simulink model "sampleModel7"  (R2021a)
settings: Solver=VariableStepAuto  StartTime=0.0  StopTime=10.0  RelTol=1e-3
undefined symbols (not defined in the file): DiscIntNeverNeededParam, magnitude, Newton, Raphson
libraries: simulink x210, pid_lib x47, simulink_need_slupdate x2
(part 1 of 8)
settings Model: Creator=user  LastModifiedBy=user

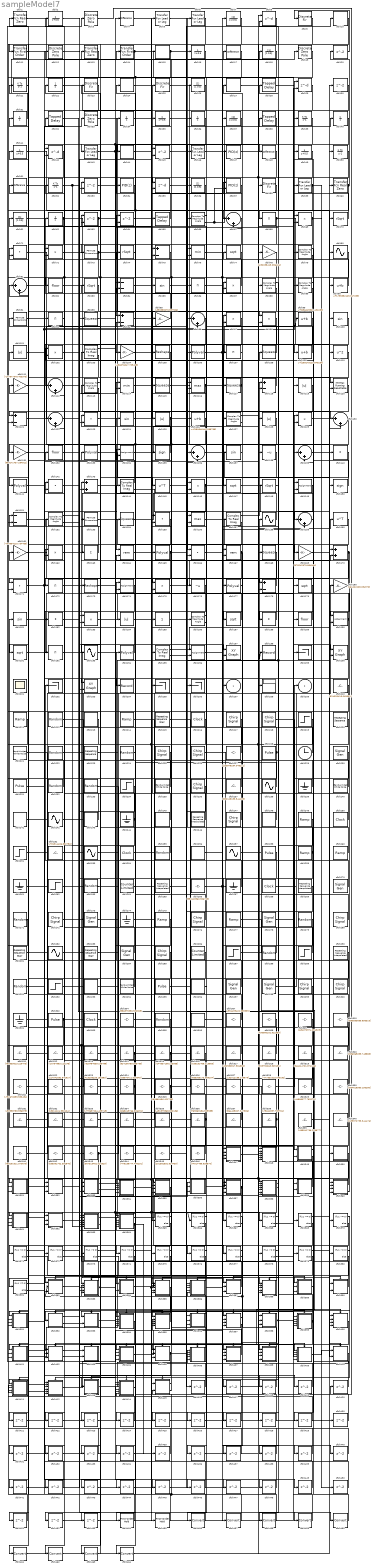
== system sampleModel7 ==
  cfblk1 : simulink/Discrete/Transfer Fcn Real Zero  ZeroZ=0.75  ICPrevInput=0.0  DoSatur=off
      settings: SourceProductBaseCode=SL
  cfblk{10,15,24,27,44} (5 alike) : DiscreteStateSpace
  cfblk{85,100,124,137,181} (5 alike) : Trigonometry
  cfblk{101,119,125,128,184} (5 alike) : Abs
  cfblk{69,98,102,162,175} (5 alike) : Product  Inputs=**
  cfblk{103,144,157,195} (4 alike) : ComplexToRealImag
  cfblk104 : Gain  Gain=[-436076047.709408]
  cfblk105 : Reshape
  cfblk{106,133,141,165,177,194} (6 alike) : Polyval  Coefs=[ +2.081618890e-019, -1.441693666e-014, +4.719686976e-010, -8.536869453e-006, +1.621573104e-001, -8.087801117e+001 ]
  cfblk{68,86,92,107,172,192} (6 alike) : Product  Inputs=*
  cfblk{93,108,115,117,154,168} (6 alike) : Squeeze
  cfblk109 : Bias  Bias=[299279220.840250]
  cfblk11 : simulink/Discrete/Transfer Fcn First Order  PoleZ=0.95  ICPrevOutput=0.0  DoSatur=off
  cfblk110 : Math  Operator=square  SaturateOnIntegerOverflow=on
  cfblk111 : Gain  Gain=[-177877978.403373]
  cfblk{67,81,96,112,122,130,136,139,159} (9 alike) : Sum  Inputs=|++
  cfblk{66,79,88..89,113,127,152,186} (8 alike) : ComplexToMagnitudeAngle
  cfblk114 : MinMax  Inputs=2
  cfblk116 : MinMax  Function=max  Inputs=2
  cfblk{75,94,118,121,178} (5 alike) : Sum  Inputs=+-
  cfblk{3,12,19,33} (4 alike) : DiscreteZeroPole  Poles=[0 0.5]  Gain=1
  cfblk120 : simulink/Math Operations/MinMax Running Resettable  Function=min  vinit=0.0
  cfblk{71,123,142,155,166,171} (6 alike) : DotProduct  InputSameDT=on  OutDataTypeStr=Inherit: Inherit via internal rule
  cfblk126 : Bias  Bias=[180646440.098758]
  cfblk{72,87,97,129,146,183} (6 alike) : Product
  cfblk13 : simulink/Discrete/Transfer Fcn Real Zero  ZeroZ=0.75  ICPrevInput=0.0  DoSatur=off
      settings: SourceProductBaseCode=SL
  cfblk131 : Gain  Gain=[934271437.284511]
  cfblk132 : Rounding
  cfblk{134,149,174,190,196} (5 alike) : Assignment  DiagnosticForDimensions=Warning  IndexOptions=Index vector (dialog)  Indices=1  OutputSizes=1
  cfblk135 : Signum
  cfblk138 : UnaryMinus
  cfblk14 : simulink/Discrete/Transfer Fcn First Order  PoleZ=0.95  ICPrevOutput=0.0  DoSatur=off
  cfblk{140,163,182,188} (4 alike) : Sum  Inputs=+
  cfblk143 : Sum
  cfblk145 : Math  Operator=transpose  SaturateOnIntegerOverflow=on
  cfblk{77,147,179,187,191} (5 alike) : Sqrt  SaturateOnIntegerOverflow=on
  cfblk{70,74,83,148} (4 alike) : Sqrt  Operator=rSqrt  AlgorithmType=Newton-Raphson  SaturateOnIntegerOverflow=on
  cfblk150 : Signum
  cfblk151 : Sum  Inputs=--
  cfblk153 : PermuteDimensions
  cfblk156 : MinMax  Function=max  Inputs=2
  cfblk158 : Sin  TimeSource=Use external signal  SampleTime=0
  cfblk{2,16,35,41,49} (5 alike) : DiscreteTransferFcn  SampleTime=1
  cfblk160 : Math  Operator=transpose  SaturateOnIntegerOverflow=on
  cfblk161 : Gain  Gain=[-744994210.734469]
  cfblk164 : Math  Operator=rem  SaturateOnIntegerOverflow=on
  cfblk167 : Math  Operator=rem  SaturateOnIntegerOverflow=on
  cfblk169 : Gain  Gain=[578242979.864904]
  cfblk{4,17,48,51} (4 alike) : simulink/Discrete/Difference  ICPrevInput=0.0  OutMin=[]  OutMax=[]  OutDataTypeStr=Inherit: Inherit via back propagation  OutDataType=fixdt(1, 16)  OutScaling=2^-10  DoSatur=off
  cfblk170 : Sum
  cfblk173 : Reshape
  cfblk176 : UnaryMinus
  cfblk{7,18,26,37,56,61} (6 alike) : DiscreteFilter  SampleTime=1
  cfblk180 : Gain  Gain=[161222208.054570]
  cfblk185 : simulink/Math Operations/Slider Gain  gain=1  low=0  high=2
  cfblk189 : Rounding
  cfblk193 : Sin  TimeSource=Use external signal  SampleTime=0
  cfblk197 : simulink/Sinks/XY Graph  xmin=-1  xmax=1  ymin=-1  ymax=1  st=-1
  cfblk198 : Record  FileSettingsInternal="{\"entries\":[{\"content\":{\"excelSettings\":{\"content\":{},\"type\":\"Streamout.ExcelSettings\"}},\"type\":\"Streamout.FileSettingStorage\",\"uuid\":\"33b5f820-dc1f-4b1a-ab87-c804d69286ae\"}],\"packageUris\":[\"http://schema.mathworks.com/mf0/streamout_blocks/R2020a\"],\"version\":\"1.0\"}"  SignalsInternal="{\"entries\":[{\"content\":{\"signals\":[{\"content\":{\"blockPath\":[\"sampleModel7/cfblk198\"],\"channel\":[],\"dimensions\":[1],\"domain\":\"samplemodel7/cfblk198\",\"lineColor\":\"#d95319\",\"plots\":[1],\"port\":1,\"sid\":[\"\"],\"signalID\":21002,\"signalName\":\"cfblk359\"},\"type\":\"RecordBlkView.Signal\",\"uuid\":\"796a8886-daab-4861-8312-900b38053f92\"}]},\"type\":\"RecordBlkView.InputSignals\",\"uuid\":\"0fedc28f-d636-42e2-b910-8174ae87f250\"}],\"packageUris\":[\"http://schema.mathworks.com/mf0/streamout_blocks/R2020a\"],\"version\":\"1.0\"}"  VisualizationBindings="{\"sparklinesplugin\":{\"info\":[{\"bindingParametersList\":[],\"subplotID\":1}]}}"
  cfblk{199,202,205..206} (4 alike) : Terminator
  cfblk{20,30,416..453} (40 alike) : Delay  SampleTime=1
  cfblk200 : simulink/Sinks/XY Graph  xmin=-1  xmax=1  ymin=-1  ymax=1  st=-1
  cfblk201 : Scope
      settings: Floating=on
  cfblk203 : simulink/Sinks/XY Graph  xmin=-1  xmax=1  ymin=-1  ymax=1  st=-1
  cfblk204 : Record  FileSettingsInternal="{\"entries\":[{\"content\":{\"excelSettings\":{\"content\":{},\"type\":\"Streamout.ExcelSettings\"}},\"type\":\"Streamout.FileSettingStorage\",\"uuid\":\"e6acbbf8-4b6b-4568-91b6-bdc9c77e83f1\"}],\"packageUris\":[\"http://schema.mathworks.com/mf0/streamout_blocks/R2020a\"],\"version\":\"1.0\"}"  SignalsInternal="{\"entries\":[{\"content\":{\"signals\":[{\"content\":{\"blockPath\":[\"sampleModel7/cfblk204\"],\"channel\":[],\"dimensions\":[1],\"domain\":\"samplemodel7/cfblk204\",\"lineColor\":\"#b746ff\",\"plots\":[1],\"port\":1,\"sid\":[\"\"],\"signalID\":21034,\"signalName\":\"cfblk26\"},\"type\":\"RecordBlkView.Signal\",\"uuid\":\"01d88a41-b529-4621-a6f8-95e57fe73dd8\"}]},\"type\":\"RecordBlkView.InputSignals\",\"uuid\":\"3bb34bcb-c099-496e-b3bc-84ef0106e8cb\"}],\"packageUris\":[\"http://schema.mathworks.com/mf0/streamout_blocks/R2020a\"],\"version\":\"1.0\"}"  VisualizationBindings="{\"sparklinesplugin\":{\"info\":[{\"bindingParametersList\":[],\"subplotID\":1}]}}"
  cfblk208 : Display
  cfblk{21,39,50,52} (4 alike) : DiscreteIntegrator  ICPrevOutput=DiscIntNeverNeededParam  ICPrevScaledInput=DiscIntNeverNeededParam
  cfblk210 : Constant  Value=[524020415.049531]  SampleTime=1
  cfblk211 : simulink/Sources/Ramp  slope=[1030.137133]  start=[45.427189]  InitialOutput=[816826.631031]
  cfblk212 : RandomNumber  Mean=[-9496.065728]  Variance=[4869.477426]  Seed=[748697780.000000]  SampleTime=0.1
  cfblk213 : simulink/Sources/Counter Free-Running  NumBits=[31.000000]  tsamp=-1
  cfblk214 : simulink/Sources/Ramp  slope=[-5450.476118]  start=[40.178251]  InitialOutput=[-351942.154890]
  cfblk215 : simulink/Sources/Repeating Sequence Stair  OutValues=[620097113.195074, 996961577.990435]  tsamp=-1  OutMin=[]  OutMax=[]  OutDataTypeStr=double  OutputDataTypeScalingMode=double  OutDataType=fixdt(0,8)  ConRadixGroup=Best Precision: Vector-wise  OutScaling=2^-12
  cfblk{216,250,254,268,303} (5 alike) : DigitalClock
  cfblk217 : simulink/Sources/Chirp Signal  f1=[743545607.434369]  T=[-343285056.387415]  f2=[305927425.208356]
  cfblk218 : simulink/Sources/Chirp Signal  f1=[-493852260.472383]  T=[857891074.645518]  f2=[-120015420.297469]
  cfblk219 : Step  Time=[26.000000]  Before=[-790798293.471162]  After=[399582314.918579]  SampleTime=0
  cfblk{22,31,34,36,40,62} (6 alike) : UnitDelay  HasFrameUpgradeWarning=on
  cfblk220 : simulink/Sources/Repeating Sequence  rep_seq_t=[0 2]  rep_seq_y=[213258458.389968, 48619559.079898]
  cfblk221 : simulink/Sources/Band-Limited White Noise  Cov=[6528417402.634652]  Ts=0.1  seed=[9893385339.000000]
  cfblk222 : RandomNumber  Mean=[59096.277871]  Variance=[64433.860844]  Seed=[883947103.000000]  SampleTime=0.1
  cfblk223 : simulink/Sources/Repeating Sequence  rep_seq_t=[0 2]  rep_seq_y=[-569792071.335092, -150840341.118165]
  cfblk224 : RandomNumber  Mean=[93987.666809]  Variance=[65814.423769]  Seed=[597783153.000000]  SampleTime=0.1
  cfblk225 : simulink/Sources/Chirp Signal  f1=[-378273320.468828]  T=[-983632335.403246]  f2=[969737135.267250]
  cfblk226 : simulink/Sources/Chirp Signal  f1=[-563170031.250757]  T=[464970760.325772]  f2=[602740179.436445]
  cfblk227 : Constant  Value=[200978294.048211]  SampleTime=1
  cfblk228 : DiscretePulseGenerator  PulseType=Time based  Amplitude=[-669665441.401893]  Period=[35025367.756640]  PulseWidth=5  PhaseDelay=[7.000000]
  cfblk229 : Clock
  cfblk{9,23,25,58} (4 alike) : DiscreteFir  SampleTime=1
  cfblk230 : SignalGenerator  Amplitude=[-992086751.304337]
  cfblk231 : DiscretePulseGenerator  PulseType=Time based  Amplitude=[984993340.582845]  Period=[36116761.892017]  PulseWidth=5  PhaseDelay=[3.000000]
  cfblk232 : UniformRandomNumber  Minimum=[-3818046436.640810]  Maximum=[5090086403.133304]  Seed=[56812594.000000]  SampleTime=0.1
  cfblk233 : UniformRandomNumber  Minimum=[-932888726.507126]  Maximum=[6609210111.863044]  Seed=[78621193.000000]  SampleTime=0.1
  cfblk234 : Step  Time=[14.000000]  Before=[-635477653.074702]  After=[674226947.834275]  SampleTime=0
  cfblk235 : simulink/Sources/Band-Limited White Noise  Cov=[491962027.885377]  Ts=0.1  seed=[1309214404.000000]
  cfblk236 : simulink/Sources/Chirp Signal  f1=[-403885962.803883]  T=[132909770.054147]  f2=[-111427795.279473]
  cfblk237 : Constant  Value=[852128153.544189]  SampleTime=1
  cfblk238 : Sin  Amplitude=[202876391.396995]  Bias=[622083626.491215]  SampleTime=0
  cfblk{239,244,261,267,274,301} (6 alike) : Ground
  cfblk240 : simulink/Sources/Band-Limited White Noise  Cov=[8151406213.355165]  Ts=0.1  seed=[616741273.000000]
  cfblk241 : simulink/Sources/Counter Free-Running  NumBits=[13.000000]  tsamp=-1
  cfblk242 : Sin  Amplitude=[-301429893.411587]  Bias=[-578206961.244922]  SampleTime=0
  cfblk243 : simulink/Sources/Counter Free-Running  NumBits=[13.000000]  tsamp=-1
  cfblk245 : simulink/Sources/Counter Free-Running  NumBits=[20.000000]  tsamp=-1
  cfblk246 : simulink/Sources/Repeating Sequence Interpolated  OutValues=[-450645048.681899, 465095687.906340, 414797516.535470, -426302903.466728, -987112265.543416]  TimeValues=[0 0.1 0.5 0.6 1].'  LookUpMeth=Use Input Nearest  tsamp=0.01  OutMin=[]  OutMax=[]  OutDataTypeStr=double  OutputDataTypeScalingMode=double  OutDataType=fixdt(0,8)  OutScaling=2^-10
  cfblk247 : simulink/Sources/Chirp Signal  f1=[-319865348.200507]  T=[-112136263.341765]  f2=[-601953811.778989]
  cfblk248 : simulink/Sources/Counter Free-Running  NumBits=[22.000000]  tsamp=-1
  cfblk249 : simulink/Sources/Ramp  slope=[4946.348764]  start=[16.631799]  InitialOutput=[956548.997204]
  cfblk251 : Step  Time=[48.000000]  Before=[695171433.417736]  After=[177666728.297122]  SampleTime=0
  cfblk252 : Constant  Value=[-781314406.882750]  SampleTime=1
  cfblk253 : Sin  Amplitude=[-11513605.676250]  Bias=[-821857418.853351]  SampleTime=0
  cfblk255 : UniformRandomNumber  Minimum=[-701801758.865852]  Maximum=[8678339802.126019]  Seed=[68934056.000000]  SampleTime=0.1
  cfblk256 : simulink/Sources/Counter Free-Running  NumBits=[19.000000]  tsamp=-1
  cfblk257 : Sin  Amplitude=[-411844016.363689]  Bias=[201928634.661419]  SampleTime=0
  cfblk258 : DiscretePulseGenerator  PulseType=Time based  Amplitude=[-474102356.549540]  Period=[30790102.267686]  PulseWidth=5  PhaseDelay=[3.000000]
  cfblk259 : simulink/Sources/Ramp  slope=[7960.944092]  start=[45.974135]  InitialOutput=[34137.177762]
  cfblk260 : simulink/Sources/Ramp  slope=[-104.563983]  start=[44.144888]  InitialOutput=[232608.767387]
  cfblk262 : Step  Time=[8.000000]  Before=[-777670275.272579]  After=[-705023258.616207]  SampleTime=0
  cfblk263 : RandomNumber  Mean=[92822.716429]  Variance=[49071.021235]  Seed=[630192977.000000]  SampleTime=0.1
  cfblk264 : simulink/Sources/Counter Limited  uplimit=[395.000000]  tsamp=-1
  cfblk265 : simulink/Sources/Repeating Sequence Interpolated  OutValues=[582550086.818798, 378877582.389652, 420436919.398782, -767860329.071510, 871635005.758899]  TimeValues=[0 0.1 0.5 0.6 1].'  LookUpMeth=Use Input Nearest  tsamp=0.01  OutMin=[]  OutMax=[]  OutDataTypeStr=double  OutputDataTypeScalingMode=double  OutDataType=fixdt(0,8)  OutScaling=2^-10
  cfblk266 : Constant  Value=[953418960.906703]  SampleTime=1
  cfblk269 : simulink/Sources/Repeating Sequence Interpolated  OutValues=[24439926.283149, -764111606.177588, 284652558.125769, -333748133.871525, 968266300.835480]  TimeValues=[0 0.1 0.5 0.6 1].'  LookUpMeth=Use Input Above  tsamp=0.01  OutMin=[]  OutMax=[]  OutDataTypeStr=double  OutputDataTypeScalingMode=double  OutDataType=fixdt(0,8)  OutScaling=2^-10
  cfblk270 : SignalGenerator  Amplitude=[894529370.076149]  Units=rad/sec
  cfblk271 : RandomNumber  Mean=[-87458.014011]  Variance=[15420.417994]  Seed=[930721984.000000]  SampleTime=0.1
  cfblk272 : simulink/Sources/Chirp Signal  f1=[-329172158.501780]  T=[-335641080.512788]  f2=[-39141377.640128]
  cfblk273 : SignalGenerator  WaveForm=square  Amplitude=[394650273.027109]  Units=rad/sec
  cfblk275 : simulink/Sources/Ramp  slope=[7083.231616]  start=[44.227960]  InitialOutput=[737333.840451]
  cfblk276 : simulink/Sources/Chirp Signal  f1=[-651584684.508423]  T=[-556322214.516704]  f2=[-126128626.986041]
  cfblk277 : simulink/Sources/Ramp  slope=[-9076.234007]  start=[31.699292]  InitialOutput=[-816121.492388]
  cfblk278 : SignalGenerator  WaveForm=square  Amplitude=[151893873.336181]
  cfblk279 : RandomNumber  Mean=[-86026.753652]  Variance=[87554.267207]  Seed=[329952460.000000]  SampleTime=0.1
  cfblk{28,32,38,65} (4 alike) : simulink/Discrete/Tapped Delay  vinit=0.0  samptime=-1  NumDelays=1  DelayOrder=Oldest  includeCurrent=off
  cfblk280 : simulink/Sources/Chirp Signal  f1=[903993729.853343]  T=[819500778.137060]  f2=[913581693.425247]
  cfblk281 : simulink/Sources/Repeating Sequence Stair  OutValues=[-518754567.655191, -580569798.246538]  tsamp=-1  OutMin=[]  OutMax=[]  OutDataTypeStr=double  OutputDataTypeScalingMode=double  OutDataType=fixdt(0,8)  ConRadixGroup=Best Precision: Vector-wise  OutScaling=2^-12
  cfblk282 : Sin  Amplitude=[5735855.369506]  Bias=[68993685.687378]  SampleTime=0
  cfblk283 : simulink/Sources/Repeating Sequence Stair  OutValues=[-908322828.357433, -917374741.295317]  tsamp=-1  OutMin=[]  OutMax=[]  OutDataTypeStr=double  OutputDataTypeScalingMode=double  OutDataType=fixdt(0,8)  ConRadixGroup=Best Precision: Vector-wise  OutScaling=2^-12
  cfblk284 : SignalGenerator  WaveForm=square  Amplitude=[526675952.966053]
  cfblk285 : simulink/Sources/Chirp Signal  f1=[193150470.797075]  T=[57635887.761176]  f2=[912894724.060447]
  cfblk286 : simulink/Sources/Counter Limited  uplimit=[404.000000]  tsamp=-1
  cfblk287 : Step  Time=[40.000000]  Before=[996055666.687662]  After=[251563225.588835]  SampleTime=0
  cfblk288 : UniformRandomNumber  Minimum=[-7496835967.641567]  Maximum=[8729181639.729187]  Seed=[5649486.000000]  SampleTime=0.1
  cfblk289 : Step  Time=[10.000000]  Before=[857137299.471670]  After=[-96536403.778174]  SampleTime=0
  cfblk{8,29,42,55} (4 alike) : Delay  DelayLengthSource=Input port  SampleTime=1
      settings: InputPortMap=u0,p1
  cfblk290 : simulink/Sources/Repeating Sequence Interpolated  OutValues=[565215223.963382, -475259355.929744, 977523137.003072, 200937123.605233, -160039889.164123]  TimeValues=[0 0.1 0.5 0.6 1].'  LookUpMeth=Use Input Above  tsamp=0.01  OutMin=[]  OutMax=[]  OutDataTypeStr=double  OutputDataTypeScalingMode=double  OutDataType=fixdt(0,8)  OutScaling=2^-10
  cfblk291 : RandomNumber  Mean=[-26763.666049]  Variance=[58579.543437]  Seed=[178776162.000000]  SampleTime=0.1
  cfblk292 : Step  Time=[30.000000]  Before=[116319489.559848]  After=[164052589.890091]  SampleTime=0
  cfblk293 : simulink/Sources/Counter Free-Running  NumBits=[21.000000]  tsamp=-1
  cfblk294 : simulink/Sources/Band-Limited White Noise  Cov=[1934120681.365680]  Ts=0.1  seed=[5475971794.000000]
  cfblk295 : DiscretePulseGenerator  PulseType=Time based  Amplitude=[596723854.655416]  Period=[36879074.032624]  PulseWidth=5  PhaseDelay=[5.000000]
  cfblk296 : simulink/Sources/Counter Free-Running  NumBits=[53.000000]  tsamp=-1
  cfblk297 : SignalGenerator  WaveForm=sawtooth  Amplitude=[656379074.653439]
  cfblk298 : SignalGenerator  Amplitude=[-439043768.529233]  Units=rad/sec
  cfblk299 : simulink/Sources/Chirp Signal  f1=[-753347408.556282]  T=[379872310.866754]  f2=[-968584085.001590]
  cfblk300 : simulink/Sources/Chirp Signal  f1=[604165645.787270]  T=[-503021265.049175]  f2=[819974698.514872]
  cfblk302 : DiscretePulseGenerator  PulseType=Time based  Amplitude=[-464926827.343680]  Period=[95246281.630336]  PulseWidth=5  PhaseDelay=[4.000000]
  cfblk304 : Constant  Value=[586575390.552825]  SampleTime=1
  cfblk305 : RandomNumber  Mean=[33528.370879]  Variance=[26957.875777]  Seed=[805936811.000000]  SampleTime=0.1
  cfblk306 : simulink/Sources/Counter Free-Running  NumBits=[53.000000]  tsamp=-1
  cfblk307 : Constant  Value=[-954439422.989939]  SampleTime=1
  cfblk308 : Constant  Value=[436080102.912559]  SampleTime=1
  cfblk309 : Constant  Value=[-634072574.054325]  SampleTime=1
  cfblk310 : Constant  Value=[-680553689.856316]  SampleTime=1
  cfblk311 : Constant  Value=[760535013.226473]  SampleTime=1
  cfblk312 : Constant  Value=[-16794983.122245]  SampleTime=1
  cfblk313 : Constant  Value=[-318484039.166498]  SampleTime=1
  cfblk314 : Constant  Value=[824106789.505750]  SampleTime=1
  cfblk315 : Constant  Value=[-244337108.123065]  SampleTime=1
  cfblk316 : Constant  Value=[-109231408.213983]  SampleTime=1
  cfblk317 : Constant  Value=[492980817.584880]  SampleTime=1
  cfblk318 : Constant  Value=[333792263.325191]  SampleTime=1
  cfblk319 : Constant  Value=[346214701.871126]  SampleTime=1
  cfblk320 : Constant  Value=[-956365099.748888]  SampleTime=1
  cfblk321 : Constant  Value=[-752670059.933454]  SampleTime=1
  cfblk322 : Constant  Value=[227041692.841627]  SampleTime=1
  cfblk323 : Constant  Value=[423295235.193383]  SampleTime=1
  cfblk324 : Constant  Value=[-35970711.013645]  SampleTime=1
  cfblk325 : Constant  Value=[-60860456.421755]  SampleTime=1
  cfblk326 : Constant  Value=[-665306173.089104]  SampleTime=1
  cfblk327 : Constant  Value=[132012188.179679]  SampleTime=1
  cfblk328 : Constant  Value=[-777531019.049252]  SampleTime=1
  cfblk329 : Constant  Value=[-44886077.763270]  SampleTime=1
  cfblk330 : Constant  Value=[-564618580.156280]  SampleTime=1
  cfblk331 : Constant  Value=[-58998783.596879]  SampleTime=1
  cfblk332 : Constant  Value=[15011124.930104]  SampleTime=1
  cfblk333 : Constant  Value=[-775637204.439745]  SampleTime=1
  cfblk334 : Constant  Value=[-868249766.306151]  SampleTime=1
  cfblk335 : Constant  Value=[-491979568.832186]  SampleTime=1
  cfblk336 : Constant  Value=[769063186.505985]  SampleTime=1
  cfblk337 : Constant  Value=[864425027.347386]  SampleTime=1
  cfblk338 : Constant  Value=[-75611897.789784]  SampleTime=1
  cfblk339 : Constant  Value=[-495541796.229877]  SampleTime=1
  cfblk340 : Constant  Value=[-159372753.344476]  SampleTime=1
  cfblk341 : Constant  Value=[765291611.070670]  SampleTime=1
  cfblk342 : Constant  Value=[635591702.392840]  SampleTime=1
  cfblk343 : Constant  Value=[367315462.010529]  SampleTime=1
  cfblk344 : Constant  Value=[-476238774.440251]  SampleTime=1
  cfblk345 : Constant  Value=[201382552.814439]  SampleTime=1
  cfblk346 : Constant  Value=[74017486.635570]  SampleTime=1
  cfblk347 : Subsystem
  cfblk348 : Subsystem
  cfblk349 : Subsystem
  cfblk350 : Subsystem
  cfblk351 : Subsystem
  cfblk352 : Subsystem
  cfblk353 : Subsystem
  cfblk354 : Subsystem
  cfblk355 : Subsystem
  cfblk356 : Subsystem
  cfblk357 : Subsystem
  cfblk358 : Subsystem
  cfblk359 : Subsystem
  cfblk360 : Subsystem
  cfblk361 : Subsystem
  cfblk362 : Subsystem
  cfblk363 : Subsystem
  cfblk364 : Subsystem
  cfblk{365..381} (17 alike) : If  IfExpression=u1 >= 0  SampleTime=1
  cfblk382 : Subsystem  TreatAsAtomicUnit=on
  cfblk383 : Subsystem  TreatAsAtomicUnit=on
  cfblk384 : Subsystem  TreatAsAtomicUnit=on
  cfblk385 : Subsystem  TreatAsAtomicUnit=on
  cfblk386 : Subsystem  TreatAsAtomicUnit=on
  cfblk387 : Subsystem  TreatAsAtomicUnit=on
  cfblk388 : Subsystem  TreatAsAtomicUnit=on
  cfblk389 : Subsystem  TreatAsAtomicUnit=on
  cfblk390 : Subsystem  TreatAsAtomicUnit=on
  cfblk391 : Subsystem  TreatAsAtomicUnit=on
  cfblk392 : Subsystem  TreatAsAtomicUnit=on
  cfblk393 : Subsystem  TreatAsAtomicUnit=on
  cfblk394 : Subsystem  TreatAsAtomicUnit=on
  cfblk395 : Subsystem  TreatAsAtomicUnit=on
  cfblk396 : Subsystem  TreatAsAtomicUnit=on
  cfblk397 : Subsystem  TreatAsAtomicUnit=on
  cfblk398 : Subsystem  TreatAsAtomicUnit=on
  cfblk399 : Subsystem  TreatAsAtomicUnit=on
  cfblk400 : Subsystem  TreatAsAtomicUnit=on
  cfblk401 : Subsystem  TreatAsAtomicUnit=on
  cfblk402 : Subsystem  TreatAsAtomicUnit=on
  cfblk403 : Subsystem  TreatAsAtomicUnit=on
  cfblk404 : Subsystem  TreatAsAtomicUnit=on
  cfblk405 : Subsystem  TreatAsAtomicUnit=on
  cfblk406 : Subsystem  TreatAsAtomicUnit=on
  cfblk407 : Subsystem  TreatAsAtomicUnit=on
  cfblk408 : Subsystem  TreatAsAtomicUnit=on
  cfblk409 : Subsystem  TreatAsAtomicUnit=on
  cfblk410 : Subsystem  TreatAsAtomicUnit=on
  cfblk411 : Subsystem  TreatAsAtomicUnit=on
  cfblk412 : Subsystem  TreatAsAtomicUnit=on
  cfblk413 : Subsystem  TreatAsAtomicUnit=on
  cfblk414 : Subsystem  TreatAsAtomicUnit=on
  cfblk415 : Subsystem  TreatAsAtomicUnit=on
  cfblk{5..6,43,46,59} (5 alike) : simulink/Discrete/Transfer Fcn Lead or Lag  PoleZ=0.95  ZeroZ=0.75  ICPrevOutput=0.0  ICPrevInput=0.0  DoSatur=off
      settings: SourceProductBaseCode=SL
  cfblk{45,53,63..64} (4 alike) : Delay  ShowEnablePort=on  SampleTime=1
      settings: InputPortMap=u0,e6
  cfblk454 : simulink_need_slupdate/First-Order Hold  DisableCoverage=on  Ts=1
      settings: SourceProductBaseCode=SL
  cfblk455 : simulink_need_slupdate/First-Order Hold  DisableCoverage=on  Ts=1
      settings: SourceProductBaseCode=SL
  cfblk{456..464} (9 alike) : DataTypeConversion
  cfblk47 : pid_lib/PID Controller  Controller=PID  Form=Parallel  TimeDomain=Discrete-time  UseExternalTs=off  SampleTime=1  IntegratorMethod=Forward Euler  FilterMethod=Forward Euler  ControllerParametersSource=internal  P=1  I=1  D=0  UseFilter=on  N=100  TunerSelectOption=Transfer Function Based (PID Tuner App)  InitialConditionSource=internal  InitialConditionForIntegrator=0  InitialConditionForFilter=0  DifferentiatorICPrevScaledInput=0  ExternalReset=none  TrackingMode=off  Kt=1  LimitOutput=off  SatLimitsSource=internal  UpperSaturationLimit=inf  LowerSaturationLimit=-inf  LinearizeAsGain=off  AntiWindupMode=none  Kb=1  POutMin=[]  POutMax=[]  IOutMin=[]  IOutMax=[]  DOutMin=[]  DOutMax=[]  NOutMin=[]  NOutMax=[]  SumOutMin=[]  SumOutMax=[]  SaturationOutMin=[]  SaturationOutMax=[]  PParamMin=[]  PParamMax=[]  IParamMin=[]  IParamMax=[]  DParamMin=[]  DParamMax=[]  NParamMin=[]  NParamMax=[]  KbParamMin=[]  KbParamMax=[]  KtParamMin=[]  KtParamMax=[]  KbOutMin=[]  KbOutMax=[]  KtOutMin=[]  KtOutMax=[]  IntegratorOutMin=[]  IntegratorOutMax=[]  FilterOutMin=[]  FilterOutMax=[]  SumI1OutMin=[]  SumI1OutMax=[]  SumI2OutMin=[]  SumI2OutMax=[]  SumI3OutMin=[]  SumI3OutMax=[]  SumI4OutMin=[]  SumI4OutMax=[]  SumDOutMin=[]  SumDOutMax=[]  DifferentiatorOutMin=[]  DifferentiatorOutMax=[]  FilterDiffOutCoefMin=[]  FilterDiffOutCoefMax=[]  ReciprocalOutMin=[]  ReciprocalOutMax=[]  SumDenOutMin=[]  SumDenOutMax=[]  SumNumOutMin=[]  SumNumOutMax=[]  DivideOutMin=[]  DivideOutMax=[]  UdiffTsProdOutMin=[]  UdiffTsProdOutMax=[]  NTsProdOutMin=[]  NTsProdOutMax=[]  UintegralTsProdOutMin=[]  UintegralTsProdOutMax=[]  UngainTsProdOutMin=[]  UngainTsProdOutMax=[]  IntegratorContinuousStateAttributes=''  IntegratorStateMustResolveToSignalObject=off  IntegratorRTWStateStorageClass=Auto  FilterContinuousStateAttributes=''  FilterStateMustResolveToSignalObject=off  FilterRTWStateStorageClass=Auto  ParallelPVariant=InternalParameters  IdealPVariant=Disabled  IVariant=InternalParameters  DVariant=InternalParameters  IntegratorVariant=Discrete  SatVariant=Disabled  AWVariant=Passthrough  PCopyVariant=Disabled  TRVariant=Disabled  FdbkBlocksVariant=Forward  IdealPFdbkVariant=Disabled  SatFdbkVariant=Disabled  DerivativeFilterVariant=ForwardEulerFilter  NVariant=InternalParameters  NCopyVariant=Disabled  FilterICVariant=InternalICsFilter  IntegratorICVariant=InternalICs  ExternalResetVariant=Disabled  TRSumVariant=Passthrough  SumFdbkVariant=Disabled  SumVariant=Sum_PID  TsampFilterVariant=InternalTs  TsampNgainVariant=Passthrough  TsampIntegralVariant=Passthrough  ExternalSaturationOutDataTypeStr=Inherit: Same as second input
  cfblk54 : pid_lib/PID Controller  Controller=PID  Form=Parallel  TimeDomain=Discrete-time  UseExternalTs=off  SampleTime=1  IntegratorMethod=Forward Euler  FilterMethod=Forward Euler  ControllerParametersSource=internal  P=1  I=1  D=0  UseFilter=on  N=100  TunerSelectOption=Transfer Function Based (PID Tuner App)  InitialConditionSource=internal  InitialConditionForIntegrator=0  InitialConditionForFilter=0  DifferentiatorICPrevScaledInput=0  ExternalReset=none  TrackingMode=off  Kt=1  LimitOutput=off  SatLimitsSource=internal  UpperSaturationLimit=inf  LowerSaturationLimit=-inf  LinearizeAsGain=off  AntiWindupMode=none  Kb=1  POutMin=[]  POutMax=[]  IOutMin=[]  IOutMax=[]  DOutMin=[]  DOutMax=[]  NOutMin=[]  NOutMax=[]  SumOutMin=[]  SumOutMax=[]  SaturationOutMin=[]  SaturationOutMax=[]  PParamMin=[]  PParamMax=[]  IParamMin=[]  IParamMax=[]  DParamMin=[]  DParamMax=[]  NParamMin=[]  NParamMax=[]  KbParamMin=[]  KbParamMax=[]  KtParamMin=[]  KtParamMax=[]  KbOutMin=[]  KbOutMax=[]  KtOutMin=[]  KtOutMax=[]  IntegratorOutMin=[]  IntegratorOutMax=[]  FilterOutMin=[]  FilterOutMax=[]  SumI1OutMin=[]  SumI1OutMax=[]  SumI2OutMin=[]  SumI2OutMax=[]  SumI3OutMin=[]  SumI3OutMax=[]  SumI4OutMin=[]  SumI4OutMax=[]  SumDOutMin=[]  SumDOutMax=[]  DifferentiatorOutMin=[]  DifferentiatorOutMax=[]  FilterDiffOutCoefMin=[]  FilterDiffOutCoefMax=[]  ReciprocalOutMin=[]  ReciprocalOutMax=[]  SumDenOutMin=[]  SumDenOutMax=[]  SumNumOutMin=[]  SumNumOutMax=[]  DivideOutMin=[]  DivideOutMax=[]  UdiffTsProdOutMin=[]  UdiffTsProdOutMax=[]  NTsProdOutMin=[]  NTsProdOutMax=[]  UintegralTsProdOutMin=[]  UintegralTsProdOutMax=[]  UngainTsProdOutMin=[]  UngainTsProdOutMax=[]  IntegratorContinuousStateAttributes=''  IntegratorStateMustResolveToSignalObject=off  IntegratorRTWStateStorageClass=Auto  FilterContinuousStateAttributes=''  FilterStateMustResolveToSignalObject=off  FilterRTWStateStorageClass=Auto  ParallelPVariant=InternalParameters  IdealPVariant=Disabled  IVariant=InternalParameters  DVariant=InternalParameters  IntegratorVariant=Discrete  SatVariant=Disabled  AWVariant=Passthrough  PCopyVariant=Disabled  TRVariant=Disabled  FdbkBlocksVariant=Forward  IdealPFdbkVariant=Disabled  SatFdbkVariant=Disabled  DerivativeFilterVariant=ForwardEulerFilter  NVariant=InternalParameters  NCopyVariant=Disabled  FilterICVariant=InternalICsFilter  IntegratorICVariant=InternalICs  ExternalResetVariant=Disabled  TRSumVariant=Passthrough  SumFdbkVariant=Disabled  SumVariant=Sum_PID  TsampFilterVariant=InternalTs  TsampNgainVariant=Passthrough  TsampIntegralVariant=Passthrough  ExternalSaturationOutDataTypeStr=Inherit: Same as second input
  cfblk57 : pid_lib/PID Controller (2DOF)  Controller=PID  Form=Parallel  TimeDomain=Discrete-time  UseExternalTs=off  SampleTime=1  IntegratorMethod=Forward Euler  FilterMethod=Forward Euler  ControllerParametersSource=internal  P=1  I=1  D=0  UseFilter=on  N=100  b=1  c=1  TunerSelectOption=Transfer Function Based (PID Tuner App)  InitialConditionSource=internal  InitialConditionForIntegrator=0  InitialConditionForFilter=0  DifferentiatorICPrevScaledInput=0  ExternalReset=none  TrackingMode=off  Kt=1  LimitOutput=off  SatLimitsSource=internal  UpperSaturationLimit=inf  LowerSaturationLimit=-inf  LinearizeAsGain=off  AntiWindupMode=none  Kb=1  POutMin=[]  POutMax=[]  IOutMin=[]  IOutMax=[]  DOutMin=[]  DOutMax=[]  NOutMin=[]  NOutMax=[]  bOutMin=[]  bOutMax=[]  cOutMin=[]  cOutMax=[]  SumOutMin=[]  SumOutMax=[]  SaturationOutMin=[]  SaturationOutMax=[]  PParamMin=[]  PParamMax=[]  IParamMin=[]  IParamMax=[]  DParamMin=[]  DParamMax=[]  NParamMin=[]  NParamMax=[]  bParamMin=[]  bParamMax=[]  cParamMin=[]  cParamMax=[]  KbParamMin=[]  KbParamMax=[]  KtParamMin=[]  KtParamMax=[]  KbOutMin=[]  KbOutMax=[]  KtOutMin=[]  KtOutMax=[]  IntegratorOutMin=[]  IntegratorOutMax=[]  FilterOutMin=[]  FilterOutMax=[]  SumI1OutMin=[]  SumI1OutMax=[]  SumI2OutMin=[]  SumI2OutMax=[]  SumI3OutMin=[]  SumI3OutMax=[]  SumI4OutMin=[]  SumI4OutMax=[]  SumDOutMin=[]  SumDOutMax=[]  Sum1OutMin=[]  Sum1OutMax=[]  Sum2OutMin=[]  Sum2OutMax=[]  Sum3OutMin=[]  Sum3OutMax=[]  DifferentiatorOutMin=[]  DifferentiatorOutMax=[]  FilterDiffOutCoefMin=[]  FilterDiffOutCoefMax=[]  ReciprocalOutMin=[]  ReciprocalOutMax=[]  SumDenOutMin=[]  SumDenOutMax=[]  SumNumOutMin=[]  SumNumOutMax=[]  DivideOutMin=[]  DivideOutMax=[]  UdiffTsProdOutMin=[]  UdiffTsProdOutMax=[]  NTsProdOutMin=[]  NTsProdOutMax=[]  UintegralTsProdOutMin=[]  UintegralTsProdOutMax=[]  UngainTsProdOutMin=[]  UngainTsProdOutMax=[]  IntegratorContinuousStateAttributes=''  IntegratorStateMustResolveToSignalObject=off  IntegratorRTWStateStorageClass=Auto  FilterContinuousStateAttributes=''  FilterStateMustResolveToSignalObject=off  FilterRTWStateStorageClass=Auto  ParallelPVariant=InternalParameters  IdealPVariant=Disabled  IVariant=InternalParameters  DVariant=InternalParameters  bVariant=InternalParameters  cVariant=InternalParameters  IntegratorVariant=Discrete  SatVariant=Disabled  AWVariant=Passthrough  PCopyVariant=Disabled  TRVariant=Disabled  FdbkBlocksVariant=Forward  IdealPFdbkVariant=Disabled  SatFdbkVariant=Disabled  DerivativeFilterVariant=ForwardEulerFilter  NVariant=InternalParameters  NCopyVariant=Disabled  FilterICVariant=InternalICsFilter  IntegratorICVariant=InternalICs  ExternalResetVariant=Disabled  TRSumVariant=Passthrough  SumFdbkVariant=Disabled  SumVariant=Sum_PID  TsampFilterVariant=InternalTs  TsampNgainVariant=Passthrough  TsampIntegralVariant=Passthrough  ExternalSaturationOutDataTypeStr=Inherit: Same as second input
      settings: SourceProductBaseCode=SL
  cfblk60 : simulink/Discrete/Transfer Fcn Real Zero  ZeroZ=0.75  ICPrevInput=0.0  DoSatur=off
      settings: SourceProductBaseCode=SL
  cfblk73 : PermuteDimensions
  cfblk76 : MinMax  Inputs=2
  cfblk78 : Gain  Gain=[-232038413.086404]
  cfblk80 : Sin  TimeSource=Use external signal  SampleTime=0
  cfblk82 : Rounding
  cfblk84 : Sum  Inputs=--
  cfblk90 : Bias  Bias=[-795352125.917099]
  cfblk91 : PermuteDimensions
  cfblk95 : Gain  Gain=[-553383073.557906]
  cfblk99 : Bias  Bias=[296219901.431288]
  cfblk207 : Outport
  cfblk209 : Outport  Port=2
  wires:
  cfblk294/1 -> cfblk194/1
  cfblk240/1 -> cfblk6/1
  cfblk238/1 -> cfblk123/1
  cfblk245/1 -> cfblk25/1
  cfblk180/1 -> cfblk129/1
  cfblk305/1 -> cfblk383/1(cfblk1), cfblk412/5(cfblk16)
  cfblk259/1 -> cfblk16/1, cfblk383/4(cfblk14)
  cfblk32/1 -> cfblk358/1(cfblk1)
  cfblk316/1 -> cfblk401/1(cfblk1)
  cfblk143/1 -> cfblk65/1
  cfblk303/1 -> cfblk377/1
  cfblk325/1 -> cfblk97/1, cfblk412/3(cfblk14)
  cfblk40/1 -> cfblk166/1
  cfblk5/1 -> cfblk206/1
  cfblk257/1 -> cfblk180/1
  cfblk66/1 -> cfblk172/1
  cfblk277/1 -> cfblk409/1(cfblk1)
  cfblk383/1(cfblk2) -> cfblk143/1, cfblk447/1
  cfblk273/1 -> cfblk365/1
  cfblk304/1 -> cfblk375/1
  cfblk21/1 -> cfblk131/1
  cfblk298/1 -> cfblk70/1
  cfblk224/1 -> cfblk24/1
  cfblk394/1(cfblk2) -> cfblk404/1(cfblk1)
  cfblk62/1 -> cfblk104/1, cfblk382/3(cfblk16)
  cfblk329/1 -> cfblk28/1
  cfblk170/1 -> cfblk190/1, cfblk357/3(cfblk11)
  cfblk364/1(cfblk2) -> cfblk160/1
  cfblk48/1 -> cfblk391/1(cfblk1)
  cfblk106/1 -> cfblk29/1, cfblk439/1
  cfblk133/1 -> cfblk145/1
  cfblk352/1(cfblk2) -> cfblk173/1
  cfblk403/1(cfblk2) -> cfblk3/1
  cfblk36/1 -> cfblk374/1
  cfblk192/1 -> cfblk387/1(cfblk1)
  cfblk77/1 -> cfblk395/1(cfblk1), cfblk362/3(cfblk9)
  cfblk270/1 -> cfblk202/1
  cfblk14/1 -> cfblk189/1, cfblk423/1
  cfblk31/1 -> cfblk14/1
  cfblk153/1 -> cfblk169/1
  cfblk410/1(cfblk2) -> cfblk406/1(cfblk1)
  cfblk37/1 -> cfblk94/1
  cfblk338/1 -> cfblk1/1, cfblk364/6(cfblk12)
  cfblk162/1 -> cfblk85/1
  cfblk65/1 -> cfblk45/1
  cfblk229/1 -> cfblk167/1
  cfblk284/1 -> cfblk53/1
  cfblk95/1 -> cfblk62/1
  cfblk334/1 -> cfblk110/1
  cfblk156/1 -> cfblk369/1
  cfblk178/1 -> cfblk133/1
  cfblk295/1 -> cfblk37/1
  cfblk107/1 -> cfblk77/1
  cfblk348/1(cfblk2) -> cfblk181/1
  cfblk71/1 -> cfblk136/1
  cfblk218/1 -> cfblk349/1(cfblk1)
  cfblk33/1 -> cfblk125/1
  cfblk272/1 -> cfblk165/1, cfblk388/3(cfblk15)
  cfblk333/1 -> cfblk405/3(cfblk7), cfblk385/3(cfblk10), cfblk355/1(cfblk1)
  cfblk120/1 -> cfblk141/1
  cfblk41/1 -> cfblk348/1(cfblk1)
  cfblk389/1(cfblk2) -> cfblk59/1
  cfblk97/1 -> cfblk147/1
  cfblk157/1 -> cfblk118/1
  cfblk255/1 -> cfblk63/1
  cfblk314/1 -> cfblk90/1, cfblk363/4(cfblk13)
  cfblk151/1 -> cfblk370/1
  cfblk86/1 -> cfblk177/1
  cfblk243/1 -> cfblk72/1
  cfblk228/1 -> cfblk152/1, cfblk385/5(cfblk12)
  cfblk99/1 -> cfblk146/1
  cfblk25/1 -> cfblk170/1
  cfblk54/1 -> cfblk183/2
  cfblk110/1 -> cfblk126/1
  cfblk346/1 -> cfblk71/1
  cfblk223/1 -> cfblk167/2
  cfblk343/1 -> cfblk56/1, cfblk351/3(cfblk11)
  cfblk317/1 -> cfblk174/1
  cfblk43/1 -> cfblk48/1, cfblk98/2
  cfblk337/1 -> cfblk151/1
  cfblk300/1 -> cfblk153/1
  cfblk59/1 -> cfblk450/1, cfblk451/1
  cfblk261/1 -> cfblk399/1(cfblk1)
  cfblk211/1 -> cfblk391/2(cfblk10)
  cfblk336/1 -> cfblk115/1, cfblk385/4(cfblk11)
  cfblk67/1 -> cfblk84/1
  cfblk244/1 -> cfblk132/1, cfblk402/1(cfblk1)
  cfblk363/1(cfblk2) -> cfblk8/1
  cfblk171/1 -> cfblk33/1, cfblk445/1
  cfblk345/1 -> cfblk46/1
  cfblk130/1 -> cfblk175/1, cfblk364/3(cfblk9)
  cfblk191/1 -> cfblk86/1
  cfblk351/1(cfblk2) -> cfblk138/1
  cfblk411/1(cfblk2) -> cfblk92/1
  cfblk186/1 -> cfblk156/1
  cfblk72/1 -> cfblk350/1(cfblk1)
  cfblk271/1 -> cfblk391/3(cfblk11)
  cfblk265/1 -> cfblk36/1
  cfblk231/1 -> cfblk372/1
  cfblk101/1 -> cfblk164/1
  cfblk301/1 -> cfblk390/1(cfblk1)
  cfblk58/1 -> cfblk73/1, cfblk424/1
  cfblk340/1 -> cfblk158/1, cfblk394/4(cfblk12)
  cfblk30/1 -> cfblk68/1
  cfblk413/1(cfblk2) -> cfblk66/1
  cfblk407/1(cfblk2) -> cfblk13/1
  cfblk154/1 -> cfblk118/2
  cfblk96/1 -> cfblk354/1(cfblk1)
  cfblk248/1 -> cfblk74/1
  cfblk92/1 -> cfblk392/1(cfblk1)
  cfblk235/1 -> cfblk101/1
  cfblk288/1 -> cfblk22/1
  cfblk388/1(cfblk2) -> cfblk113/1
  cfblk189/1 -> cfblk188/1
  cfblk26/1 -> cfblk204/1
  cfblk60/1 -> cfblk20/1, cfblk357/4(cfblk12)
  cfblk187/1 -> cfblk174/2
  cfblk70/1 -> cfblk49/1
  cfblk144/1 -> cfblk51/1
  cfblk165/1 -> cfblk96/1, cfblk364/5(cfblk11)
  cfblk140/1 -> cfblk393/1(cfblk1)
  cfblk274/1 -> cfblk26/1
  cfblk318/1 -> cfblk41/1
  cfblk142/1 -> cfblk108/1
  cfblk49/1 -> cfblk55/1
  cfblk384/1(cfblk2) -> cfblk139/1
  cfblk398/1(cfblk2) -> cfblk119/1, cfblk427/1
  cfblk9/1 -> cfblk151/2
  cfblk1/1 -> cfblk386/1(cfblk1)
  cfblk105/1 -> cfblk361/1(cfblk1)
  cfblk174/1 -> cfblk393/2(cfblk10)
  cfblk280/1 -> cfblk107/1
  cfblk263/1 -> cfblk387/2(cfblk6)
  cfblk176/1 -> cfblk192/1
  cfblk278/1 -> cfblk29/2
  cfblk341/1 -> cfblk53/2
  cfblk276/1 -> cfblk164/2
  cfblk215/1 -> cfblk358/2(cfblk8)
  cfblk148/1 -> cfblk178/1
  cfblk76/1 -> cfblk109/1
  cfblk258/1 -> cfblk367/1
  cfblk250/1 -> cfblk144/1
  cfblk330/1 -> cfblk2/1
  cfblk401/1(cfblk2) -> cfblk179/1
  cfblk283/1 -> cfblk407/1(cfblk1)
  cfblk193/1 -> cfblk368/1
  cfblk275/1 -> cfblk404/2(cfblk7)
  cfblk79/1 -> cfblk355/2(cfblk10)
  cfblk414/1(cfblk2) -> cfblk134/1
  cfblk122/1 -> cfblk114/1
  cfblk349/1(cfblk2) -> cfblk394/1(cfblk1)
  cfblk167/1 -> cfblk187/1, cfblk354/5(cfblk17)
  cfblk391/1(cfblk2) -> cfblk64/1, cfblk99/1
  cfblk69/1 -> cfblk412/2(cfblk13), cfblk430/1
  cfblk321/1 -> cfblk414/1(cfblk1)
  cfblk347/1(cfblk2) -> cfblk69/1
  cfblk38/1 -> cfblk404/3(cfblk8)
  cfblk168/1 -> cfblk387/3(cfblk7)
  cfblk415/1(cfblk2) -> cfblk155/1
  cfblk108/1 -> cfblk61/1
  cfblk15/1 -> cfblk120/1, cfblk361/3(cfblk11)
  cfblk183/1 -> cfblk39/1
  cfblk85/1 -> cfblk98/1
  cfblk6/1 -> cfblk11/1
  cfblk186/2 -> cfblk103/1
  cfblk126/1 -> cfblk371/1
  cfblk45/1 -> cfblk186/1
  cfblk132/1 -> cfblk45/2
  cfblk188/1 -> cfblk27/1
  cfblk297/1 -> cfblk21/1
  cfblk237/1 -> cfblk142/1
  cfblk266/1 -> cfblk97/2, cfblk408/4(cfblk8)
  cfblk39/1 -> cfblk42/2, cfblk384/2(cfblk15)
  cfblk137/1 -> cfblk87/1
  cfblk66/2 -> cfblk40/1, cfblk57/2
  cfblk363/2(cfblk16) -> cfblk91/1
  cfblk179/1 -> cfblk359/2(cfblk7)
  cfblk7/1 -> cfblk193/1
  cfblk139/1 -> cfblk80/1
  cfblk221/1 -> cfblk353/1(cfblk1)
  cfblk400/1(cfblk2) -> cfblk407/2(cfblk12)
  cfblk212/1 -> cfblk348/2(cfblk9)
  cfblk12/1 -> cfblk67/1
  cfblk360/1(cfblk2) -> cfblk12/1
  cfblk18/1 -> cfblk87/2
  cfblk134/1 -> cfblk58/1
  cfblk339/1 -> cfblk360/1(cfblk1)
  cfblk292/1 -> cfblk347/1(cfblk1)
  cfblk222/1 -> cfblk105/1
  cfblk392/1(cfblk2) -> cfblk356/1(cfblk1)
  cfblk152/1 -> cfblk197/1
  cfblk401/2(cfblk17) -> cfblk19/1
  cfblk47/1 -> cfblk129/2
  cfblk82/1 -> cfblk349/2(cfblk13)
  cfblk131/1 -> cfblk96/2
  cfblk190/1 -> cfblk135/1, cfblk363/5(cfblk14)
  cfblk356/1(cfblk2) -> cfblk360/2(cfblk8)
  cfblk393/1(cfblk2) -> cfblk170/2
  cfblk177/1 -> cfblk357/1(cfblk1)
  cfblk254/1 -> cfblk128/1
  cfblk362/1(cfblk2) -> cfblk207/1
  cfblk210/1 -> cfblk391/4(cfblk12)
  cfblk147/1 -> cfblk380/1
  cfblk282/1 -> cfblk396/1(cfblk1)
  cfblk307/1 -> cfblk161/1
  cfblk53/1 -> cfblk34/1
  cfblk296/1 -> cfblk456/1
  cfblk116/1 -> cfblk396/2(cfblk7), cfblk408/3(cfblk7)
  cfblk267/1 -> cfblk163/1
  cfblk320/1 -> cfblk35/1
  cfblk173/1 -> cfblk385/1(cfblk1)
  cfblk396/1(cfblk2) -> cfblk124/1
  cfblk29/1 -> cfblk82/1
  cfblk63/1 -> cfblk191/1, cfblk388/2(cfblk14)
  cfblk402/1(cfblk2) -> cfblk363/2(cfblk11)
  cfblk109/1 -> cfblk84/2
  cfblk182/1 -> cfblk94/2
  cfblk118/1 -> cfblk76/1
  cfblk169/1 -> cfblk60/1
  cfblk23/1 -> cfblk352/2(cfblk8)
  cfblk84/1 -> cfblk130/1
  cfblk230/1 -> cfblk399/2(cfblk11)
  cfblk129/1 -> cfblk400/1(cfblk1)
  cfblk342/1 -> cfblk414/2(cfblk9)
  cfblk64/1 -> cfblk397/1(cfblk1)
  cfblk311/1 -> cfblk117/1
  cfblk412/1(cfblk2) -> cfblk395/2(cfblk8)
  cfblk358/2(cfblk14) -> cfblk64/2
  cfblk290/1 -> cfblk381/1
  cfblk88/2 -> cfblk171/1
  cfblk44/1 -> cfblk360/4(cfblk10)
  cfblk172/1 -> cfblk106/1
  cfblk121/1 -> cfblk38/1
  cfblk98/1 -> cfblk166/2
  cfblk260/1 -> cfblk75/1
  cfblk80/1 -> cfblk421/1, cfblk422/1, cfblk203/1
  cfblk232/1 -> cfblk111/1
  cfblk405/1(cfblk2) -> cfblk10/1, cfblk442/1
  cfblk175/1 -> cfblk88/1
  cfblk100/1 -> cfblk112/1
  cfblk404/1(cfblk2) -> cfblk127/1
  cfblk61/1 -> cfblk203/2
  cfblk125/1 -> cfblk443/1, cfblk444/1, cfblk17/1
  cfblk185/1 -> cfblk136/2
  cfblk357/1(cfblk2) -> cfblk197/2, cfblk412/6(cfblk17)
  cfblk227/1 -> cfblk95/1
  cfblk68/1 -> cfblk190/2, cfblk354/4(cfblk16)
  cfblk415/2(cfblk15) -> cfblk75/2
  cfblk262/1 -> cfblk400/2(cfblk11), cfblk388/4(cfblk16)
  cfblk28/1 -> cfblk200/1
  cfblk91/1 -> cfblk352/3(cfblk9)
  cfblk359/1(cfblk2) -> cfblk198/1, cfblk157/1
  cfblk158/1 -> cfblk67/2
  cfblk128/1 -> cfblk362/2(cfblk8)
  cfblk163/1 -> cfblk71/2
  cfblk354/1(cfblk2) -> cfblk89/1
  cfblk291/1 -> cfblk122/1
  cfblk268/1 -> cfblk140/1
  cfblk310/1 -> cfblk168/1, cfblk383/3(cfblk13)
  cfblk302/1 -> cfblk195/1, cfblk412/4(cfblk15)
  cfblk22/1 -> cfblk205/1
  cfblk242/1 -> cfblk5/1
  cfblk382/1(cfblk2) -> cfblk93/1
  cfblk328/1 -> cfblk209/1
  cfblk11/1 -> cfblk176/1
  cfblk252/1 -> cfblk347/2(cfblk12)
  cfblk111/1 -> cfblk354/2(cfblk14)
  cfblk194/1 -> cfblk112/2
  cfblk387/1(cfblk2) -> cfblk155/2
  cfblk312/1 -> cfblk15/1
  cfblk285/1 -> cfblk364/1(cfblk1)
  cfblk87/1 -> cfblk23/1
  cfblk89/1 -> cfblk404/4(cfblk9)
  cfblk144/2 -> cfblk398/2(cfblk7)
  cfblk51/1 -> cfblk150/1
  cfblk46/1 -> cfblk199/1
  cfblk2/1 -> cfblk143/2
  cfblk195/1 -> cfblk120/2
  cfblk161/1 -> cfblk363/3(cfblk12)
  cfblk313/1 -> cfblk407/3(cfblk13)
  cfblk249/1 -> cfblk408/1(cfblk1)
  cfblk322/1 -> cfblk47/1
  cfblk152/2 -> cfblk44/1
  cfblk385/1(cfblk2) -> cfblk414/4(cfblk11)
  cfblk251/1 -> cfblk347/3(cfblk13)
  cfblk115/1 -> cfblk208/1
  cfblk353/1(cfblk2) -> cfblk4/1
  cfblk399/1(cfblk2) -> cfblk196/1, cfblk402/3(cfblk11)
  cfblk93/1 -> cfblk358/3(cfblk9)
  cfblk19/1 -> cfblk43/1
  cfblk326/1 -> cfblk379/1
  cfblk150/1 -> cfblk102/1
  cfblk57/1 -> cfblk171/2
  cfblk50/1 -> cfblk142/2, cfblk398/3(cfblk8)
  cfblk135/1 -> cfblk83/1
  cfblk114/1 -> cfblk389/1(cfblk1)
  cfblk103/1 -> cfblk354/3(cfblk15)
  cfblk406/1(cfblk2) -> cfblk353/2(cfblk9)
  cfblk90/1 -> cfblk32/1
  cfblk104/1 -> cfblk116/1
  cfblk136/1 -> cfblk400/3(cfblk12)
  cfblk56/1 -> cfblk121/1
  cfblk145/1 -> cfblk146/2
  cfblk181/1 -> cfblk137/1
  cfblk309/1 -> cfblk405/1(cfblk1)
  cfblk89/2 -> cfblk394/2(cfblk10)
  cfblk127/2 -> cfblk72/2
  cfblk225/1 -> cfblk401/2(cfblk15)
  cfblk247/1 -> cfblk116/2
  cfblk315/1 -> cfblk395/3(cfblk9), cfblk348/5(cfblk12)
  cfblk327/1 -> cfblk390/2(cfblk12)
  cfblk79/2 -> cfblk347/4(cfblk14), cfblk436/1
  cfblk409/1(cfblk2) -> cfblk410/1(cfblk1)
  cfblk279/1 -> cfblk397/3(cfblk8)
  cfblk219/1 -> cfblk395/4(cfblk10), cfblk411/5(cfblk16), cfblk388/5(cfblk17)
  cfblk141/1 -> cfblk356/2(cfblk9)
  cfblk220/1 -> cfblk410/2(cfblk7)
  cfblk241/1 -> cfblk148/1
  cfblk287/1 -> cfblk130/2
  cfblk364/2(cfblk13) -> cfblk432/1, cfblk435/1
  cfblk332/1 -> cfblk405/2(cfblk6)
  cfblk299/1 -> cfblk386/4(cfblk14)
  cfblk195/2 -> cfblk356/3(cfblk10)
  cfblk408/1(cfblk2) -> cfblk55/2, cfblk382/2(cfblk15)
  cfblk233/1 -> cfblk389/3(cfblk10)
  cfblk386/1(cfblk2) -> cfblk54/1
  cfblk234/1 -> cfblk353/3(cfblk10)
  cfblk24/1 -> cfblk18/1
  cfblk42/1 -> cfblk351/1(cfblk1)
  cfblk73/1 -> cfblk184/1, cfblk361/4(cfblk12)
  cfblk360/2(cfblk11) -> cfblk178/2
  cfblk323/1 -> cfblk388/1(cfblk1)
  cfblk253/1 -> cfblk30/1
  cfblk395/1(cfblk2) -> cfblk364/2(cfblk8)
  cfblk331/1 -> cfblk409/2(cfblk13)
  cfblk117/1 -> cfblk102/2, cfblk397/4(cfblk9)
  cfblk52/1 -> cfblk69/2, cfblk363/6(cfblk15)
  cfblk81/1 -> cfblk154/1
  cfblk16/1 -> cfblk384/1(cfblk1), cfblk182/1
  cfblk35/1 -> cfblk76/2
  cfblk335/1 -> cfblk399/3(cfblk12)
  cfblk355/1(cfblk2) -> cfblk361/2(cfblk10), cfblk394/5(cfblk13)
  cfblk392/2(cfblk7) -> cfblk123/2
  cfblk20/1 -> cfblk9/1
  cfblk358/3(cfblk15) -> cfblk394/3(cfblk11)
  cfblk397/2(cfblk10) -> cfblk413/1(cfblk1)
  cfblk17/1 -> cfblk376/1
  cfblk308/1 -> cfblk401/3(cfblk16)
  cfblk264/1 -> cfblk399/4(cfblk13)
  cfblk4/1 -> cfblk399/5(cfblk14), cfblk366/1
  cfblk83/1 -> cfblk411/1(cfblk1)
  cfblk164/1 -> cfblk57/1
  cfblk34/1 -> cfblk357/2(cfblk10)
  cfblk289/1 -> cfblk162/1
  cfblk196/1 -> cfblk200/2
  cfblk390/1(cfblk2) -> cfblk79/1
  cfblk344/1 -> cfblk385/2(cfblk9)
  cfblk138/1 -> cfblk408/2(cfblk6)
  cfblk146/1 -> cfblk396/3(cfblk8), cfblk159/2
  cfblk103/2 -> cfblk162/2
  cfblk236/1 -> cfblk406/4(cfblk6)
  cfblk216/1 -> cfblk355/4(cfblk12)
  cfblk269/1 -> cfblk406/5(cfblk7)
  cfblk113/2 -> cfblk382/1(cfblk1)
  cfblk13/1 -> cfblk121/2
  cfblk353/2(cfblk11) -> cfblk114/2
  cfblk361/2(cfblk13) -> cfblk31/1
  cfblk159/1 -> cfblk139/2
  cfblk386/2(cfblk16) -> cfblk7/1
  cfblk324/1 -> cfblk52/1, cfblk364/4(cfblk10)
  cfblk8/1 -> cfblk348/3(cfblk10)
  cfblk246/1 -> cfblk185/1
  cfblk94/1 -> cfblk196/2
  cfblk239/1 -> cfblk122/2
  cfblk102/1 -> cfblk409/3(cfblk14)
  cfblk214/1 -> cfblk400/4(cfblk13)
  cfblk27/1 -> cfblk159/1
  cfblk256/1 -> cfblk407/4(cfblk14)
  cfblk226/1 -> cfblk409/4(cfblk15)
  cfblk217/1 -> cfblk351/2(cfblk10)
  cfblk402/2(cfblk12) -> cfblk414/5(cfblk12)
  cfblk386/3(cfblk17) -> cfblk383/2(cfblk12)
  cfblk365/1 -> cfblk382/Action
  cfblk365/2 -> cfblk383/Action
  cfblk366/1 -> cfblk384/Action
  cfblk366/2 -> cfblk385/Action
  cfblk367/1 -> cfblk386/Action
  cfblk367/2 -> cfblk387/Action
  cfblk368/1 -> cfblk388/Action
  cfblk368/2 -> cfblk389/Action
  cfblk369/1 -> cfblk390/Action
  cfblk369/2 -> cfblk391/Action
  cfblk370/1 -> cfblk392/Action
  cfblk370/2 -> cfblk393/Action
  cfblk371/1 -> cfblk394/Action
  cfblk371/2 -> cfblk395/Action
  cfblk372/1 -> cfblk396/Action
  cfblk372/2 -> cfblk397/Action
  cfblk373/1 -> cfblk398/Action
  cfblk373/2 -> cfblk399/Action
  cfblk374/1 -> cfblk400/Action
  cfblk374/2 -> cfblk401/Action
  cfblk375/1 -> cfblk402/Action
  cfblk375/2 -> cfblk403/Action
  cfblk376/1 -> cfblk404/Action
  cfblk376/2 -> cfblk405/Action
  cfblk377/1 -> cfblk406/Action
  cfblk377/2 -> cfblk407/Action
  cfblk378/1 -> cfblk408/Action
  cfblk378/2 -> cfblk409/Action
  cfblk379/1 -> cfblk410/Action
  cfblk379/2 -> cfblk411/Action
  cfblk380/1 -> cfblk412/Action
  cfblk380/2 -> cfblk413/Action
  cfblk381/1 -> cfblk414/Action
  cfblk381/2 -> cfblk415/Action
  cfblk55/1 -> cfblk416/1
  cfblk416/1 -> cfblk386/2(cfblk12)
  cfblk358/1(cfblk2) -> cfblk417/1
  cfblk417/1 -> cfblk378/1
  cfblk184/1 -> cfblk418/1
  cfblk418/1 -> cfblk406/2(cfblk4)
  cfblk361/1(cfblk2) -> cfblk419/1
  cfblk419/1 -> cfblk403/1(cfblk1)
  cfblk3/1 -> cfblk420/1
  cfblk420/1 -> cfblk358/4(cfblk10)
  cfblk421/1 -> cfblk402/2(cfblk10)
  cfblk422/1 -> cfblk358/6(cfblk12)
  cfblk423/1 -> cfblk409/5(cfblk16)
  cfblk424/1 -> cfblk411/4(cfblk15)
  cfblk88/1 -> cfblk425/1
  cfblk425/1 -> cfblk398/1(cfblk1)
  cfblk119/1 -> cfblk426/1
  cfblk426/1 -> cfblk360/3(cfblk9)
  cfblk427/1 -> cfblk383/5(cfblk15)
  cfblk127/1 -> cfblk428/1
  cfblk428/1 -> cfblk363/1(cfblk1)
  cfblk350/1(cfblk2) -> cfblk429/1
  cfblk429/1 -> cfblk414/3(cfblk10)
  cfblk430/1 -> cfblk8/2
  cfblk160/1 -> cfblk431/1
  cfblk431/1 -> cfblk175/2
  cfblk432/1 -> cfblk415/1(cfblk1)
  cfblk155/1 -> cfblk433/1
  cfblk433/1 -> cfblk352/1(cfblk1)
  cfblk75/1 -> cfblk434/1
  cfblk434/1 -> cfblk395/5(cfblk11)
  cfblk435/1 -> cfblk411/3(cfblk14)
  cfblk436/1 -> cfblk358/5(cfblk11)
  cfblk397/1(cfblk2) -> cfblk437/1
  cfblk437/1 -> cfblk373/1
  cfblk349/2(cfblk14) -> cfblk438/1
  cfblk438/1 -> cfblk386/5(cfblk15)
  cfblk439/1 -> cfblk414/6(cfblk13)
  cfblk166/1 -> cfblk440/1
  cfblk440/1 -> cfblk397/2(cfblk7)
  cfblk10/1 -> cfblk441/1
  cfblk441/1 -> cfblk403/2(cfblk10)
  cfblk442/1 -> cfblk412/1(cfblk1)
  cfblk443/1 -> cfblk156/2
  cfblk444/1 -> cfblk348/6(cfblk13)
  cfblk445/1 -> cfblk348/4(cfblk11)
  cfblk124/1 -> cfblk446/1
  cfblk446/1 -> cfblk183/1
  cfblk447/1 -> cfblk358/7(cfblk13)
  cfblk123/1 -> cfblk448/1
  cfblk448/1 -> cfblk386/3(cfblk13)
  cfblk411/2(cfblk17) -> cfblk449/1
  cfblk449/1 -> cfblk406/3(cfblk5)
  cfblk450/1 -> cfblk42/1
  cfblk451/1 -> cfblk411/2(cfblk13)
  cfblk113/1 -> cfblk452/1
  cfblk452/1 -> cfblk389/2(cfblk9)
  cfblk157/2 -> cfblk453/1
  cfblk453/1 -> cfblk359/1(cfblk1)
  cfblk319/1 -> cfblk454/1
  cfblk454/1 -> cfblk81/1
  cfblk281/1 -> cfblk455/1
  cfblk455/1 -> cfblk81/2
  cfblk456/1 -> cfblk415/2(cfblk14), cfblk355/3(cfblk11)
  cfblk306/1 -> cfblk457/1
  cfblk457/1 -> cfblk134/2
  cfblk149/1 -> cfblk458/1
  cfblk458/1 -> cfblk362/1(cfblk1)
  cfblk293/1 -> cfblk459/1
  cfblk459/1 -> cfblk149/1
  cfblk112/1 -> cfblk460/1
  cfblk460/1 -> cfblk149/2
  cfblk286/1 -> cfblk461/1
  cfblk461/1 -> cfblk100/1
  cfblk213/1 -> cfblk462/1
  cfblk462/1 -> cfblk50/1
  cfblk78/1 -> cfblk463/1
  cfblk463/1 -> cfblk63/2
  cfblk74/1 -> cfblk464/1
  cfblk464/1 -> cfblk78/1
